simulink model "quadrotor_r2022b"  (R2022b)
settings: Solver=ode4  StartTime=0.0  StopTime=60  FixedStep=1e-3  RelTol=1e-3
libraries: slpidlib x10, dspindex x6, sharedtransform x3, simulink x3, shared6dof x1
(part 1 of 2)
Description:
  | 22
settings Model: Creator=vplus  LastModifiedBy=vplus

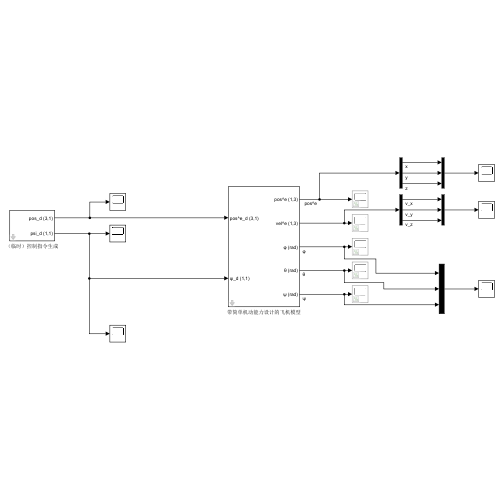
[thumbnail: Simulink's stored preview of the top-level diagram]
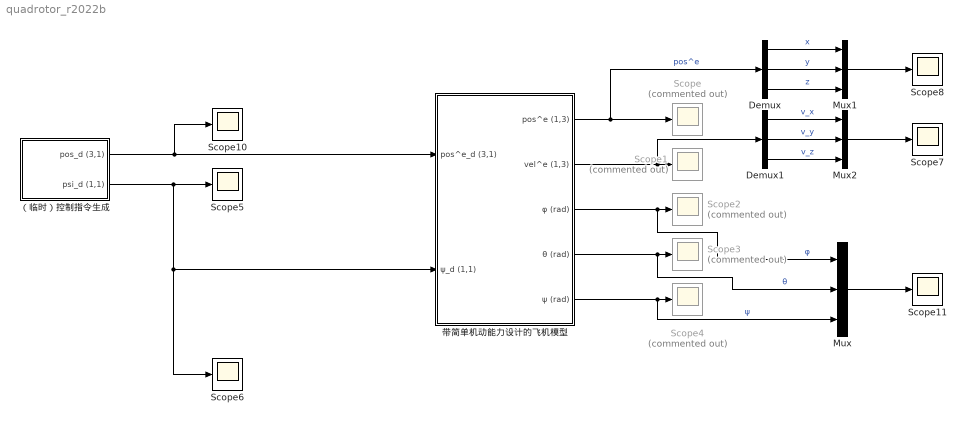
== system quadrotor_r2022b ==
  Demux : Demux  Outputs=3
  Demux1 : Demux  Outputs=3
  Mux : Mux  Inputs=3
  Mux1 : Mux  Inputs=3
  Mux2 : Mux  Inputs=3
  Scope{,1..4} (5 alike) : Scope  Commented=on
  Scope{5..8,10..11} (6 alike) : Scope
  带简单机动能力设计的飞机模型 : Subsystem  mask{Delta_t_theta=2.0, alpha_G=0.01, beta_G=0.5, rotor_w_max_rpm=240, n_rotors=4, g=9.8, mass=1.0, innertia=eye(3)}
      mask prompts: Delta_t_theta "转90° 预期时间 Δt_θ (s)"; alpha_G "α_G"; beta_G "β_G"; rotor_w_max_rpm "单发最大转速 ω_max (r/min)"; n_rotors "旋翼个数 n"; g "重力加速度 g (m/s^2)"; mass "质量 m (kg)"; innertia "转动惯量矩阵 I (kg*m^2)"
      mask init:
      | rpm2radps = (2*pi/60);
      | rotor_w_max = rotor_w_max_rpm*rpm2radps
      | % 拉力
      | f_max = (1+beta_G)*(mass*g);
      | C_T = f_max/(n_rotors* rotor_w_max^2)
      | rotor_w_min = rotor_w_max* sqrt((1-alpha_G)/(1+beta_G))
      | rotor_w_min_rpm = rotor_w_min/rpm2radps
      | 
      | % 角速度限制
      | dot_omega_z_max = 4*(pi/2)/(Delta_t_theta^2);
      | tau_z_max = abs(innertia(3,3)*dot_omega_z_max)
      | 
      | % 扭矩
      | C_M = tau_z_max/(2*(rotor_w_max^2-rotor_w_min^2))
      mask DialogControl ParameterGroupVar Prompt: 参数
      mask DialogControl Container3 Prompt: 拉力系数计算
  （临时）控制指令生成 : Subsystem  mask{rpy_0=[0,0,0], pos_0=[10,30,-2], vel_0=[1,1,0], a_h_max=1e-2, a_z_max=1e-3}
      mask prompts: rpy_0 "初始欧拉角 [φ,θ,ψ]_d (1,3) rad"; pos_0 "初始位置 p^e_d (1,3) (m/s)"; vel_0 "初始速度 v^e_d (1,3) (m/s)"; a_h_max "横向加速度最大值 a_h_max"; a_z_max "纵向加速度最大值 a_z_max"
      mask DialogControl ParameterGroupVar Prompt: 参数
  wires:
  Demux/1 -> Mux1/1  "x"
  Demux/3 -> Mux1/3  "z"
  Demux/2 -> Mux1/2  "y"
  （临时）控制指令生成/2(psi_d (1,1)) -> Scope5/1, 带简单机动能力设计的飞机模型/2("ψ_d (1,1) "), Scope6/1
  （临时）控制指令生成/1(pos_d (3,1)) -> 带简单机动能力设计的飞机模型/1(pos^e_d (3,1)), Scope10/1
  带简单机动能力设计的飞机模型/1(pos^e (1,3)) -> Demux/1, Scope/1  "pos^e"
  带简单机动能力设计的飞机模型/3(φ (rad)) -> Mux/1, Scope2/1  "φ"
  带简单机动能力设计的飞机模型/4(θ (rad)) -> Mux/2, Scope3/1  "θ"
  带简单机动能力设计的飞机模型/5(ψ (rad)) -> Mux/3, Scope4/1  "ψ"
  Mux/1 -> Scope11/1
  Mux1/1 -> Scope8/1
  Demux1/3 -> Mux2/3  "v_z"
  Mux2/1 -> Scope7/1
  带简单机动能力设计的飞机模型/2(vel^e (1,3)) -> Demux1/1, Scope1/1
  Demux1/2 -> Mux2/2  "v_y"
  Demux1/1 -> Mux2/1  "v_x"

== system quadrotor_r2022b/带简单机动能力设计的飞机模型 ==
  pos^e_d (3,1) : Inport
  "ψ_d (1,1) " : Inport  Port=2
  四旋翼无人机 : Subsystem  mask{mass=mass, innertia=innertia, g=g, C_T=C_T, C_M=C_M, L=0.2, w_max_rpm=rotor_w_max_rpm, w_min_rpm=rotor_w_min_rpm, pos_0_e=[0,0,0], vel_0_e=[0,0,0], rpy_0=[0,0,0], omega_0_b=[0,0,0], w_0=rotor_w_min*ones(1,4)}
      mask prompts: mass "质量 m (kg)"; innertia "体轴系转动惯量 I^b (kg*m^2)"; g "重力加速度 g  (m/s^2)"; C_T "旋翼拉力系数 C_T  (|T_i|=C_T*w_i^2)"; C_M "旋翼扭矩系数 C_M  (|M_i|=C_M*w_i^2)"; L "转子到体轴系原点的距离 L (m)"; w_max_rpm "旋翼最大转速 (r/min)"; w_min_rpm "旋翼最小转速 (r/min)"; pos_0_e "初始ned位置 p_0 (1,3) m"; vel_0_e "初始ned速度 v_0 (1,3) m/s"; rpy_0 "初始欧拉角 [φ,θ,ψ] (1,3) rad"; omega_0_b "初始角速度 ω^b (1,3) rad/s"; w_0 "初始旋翼转速 w (1,4) rad/s"
      mask init:
      | rpm2radps = 2*pi/60;
      | rotor_w_max = w_max_rpm *rpm2radps;
      | rotor_w_min = w_min_rpm *rpm2radps;
      | 
      | g_b = [0,0,1];
      | e_g_b = (g_b(:)/norm(g_b)); % 体轴系的重力方向,(3,1)
      | 
      | rotors_dir = [1,-1,1,-1];%旋翼的旋转方向(与体轴系Z同向记为正)
      | rotors_pos_b = [
      |     -1,-1,0;
      |     -1,1,0;
      |     1,1,0;
      |     1,-1,0
      | ]*L;% 四个旋翼的体轴系位置
      | 
      | rotors_dir=sign(rotors_dir(:)); % (n,1)
      | rotors_n = size(rotors_pos_b,1); % 电机数量
      | omegas=rotors_dir*(e_g_b'); % (n,3) 旋翼组的角速度朝向(右手定则,与重力同向为正)
      | 
      | assert(all(size(rotors_pos_b)==[rotors_n,3]),"旋翼相对位置格式错误")
      | assert(all(size(rotors_dir)==[rotors_n,1]),"旋翼旋转方向格式错误")
      | assert(all(size(e_g_b)==[3,1]),"重力方向尺寸错误")
      | 
      | f_max = rotors_n*C_T*(rotor_w_max^2); % 最大拉力
      | f_min = rotors_n*C_T*(rotor_w_min^2); % 最小拉力
      | mat_control=zeros(4,rotors_n); % [T,tau]=M*ws
      | for i=1:rotors_n
      | 
      |     r_i = rotors_pos_b(i,:);
      |     c_T_i = C_T*-e_g_b';
      | 
      |     c_MT_i = cross(r_i,c_T_i);
      |     c_MR_i = -C_M*omegas(i,:);
      |     c_M_i = c_MT_i + c_MR_i;
      |     for k=1:4
      |         if k==1
      |             mat_control(k,i) = -c_T_i(3);
      |         else
      |             mat_control(k,i) = c_M_i(k-1);
      |         end
      |     end
      | end
      | mat_control_inv = inv(mat_control);
      mask DialogControl DescTextVar Prompt: 体轴系为NED体轴系
      mask DialogControl ParameterGroupVar Prompt: 参数
      mask DialogControl Container3 Prompt: 初始状态
  pos^e (1,3) : Outport
  vel^e (1,3) : Outport  Port=2
  φ (rad) : Outport  Port=3
  θ (rad) : Outport  Port=4
  ψ (rad) : Outport  Port=5
  wires:
  "ψ_d (1,1) "/1 -> 四旋翼无人机/2("ψ_d (1,1) ")
  pos^e_d (3,1)/1 -> 四旋翼无人机/1(pos^e_d (3,1))
  四旋翼无人机/1(pos^e (1,3)) -> pos^e (1,3)/1  "pos^e"
  四旋翼无人机/2(vel^e (1,3)) -> vel^e (1,3)/1
  四旋翼无人机/3(φ (rad)) -> φ (rad)/1  "φ"
  四旋翼无人机/5(ψ (rad)) -> ψ (rad)/1  "ψ"
  四旋翼无人机/4(θ (rad)) -> θ (rad)/1  "θ"

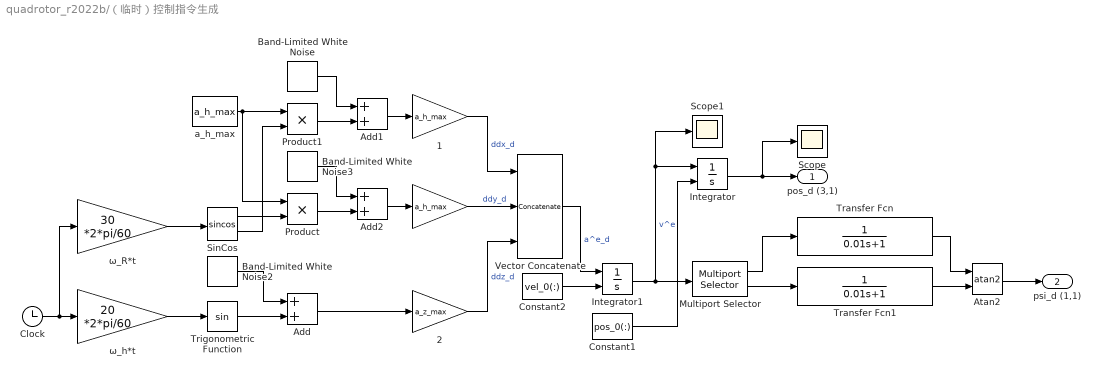
== system quadrotor_r2022b/（临时）控制指令生成 ==
  " " : Gain  Gain=a_h_max
  " 1" : Gain  Gain=a_h_max
  " 2" : Gain  Gain=a_z_max
  Add : Sum
  Add1 : Sum
  Add2 : Sum
  Atan2 : Trigonometry  Operator=atan2
  Band-Limited White Noise : simulink/Sources/Band-Limited White Noise  Cov=0.1  Ts=0.1  seed=[randi(10086)]
  Band-Limited White Noise2 : simulink/Sources/Band-Limited White Noise  Cov=0.1  Ts=0.1  seed=[randi(10086)]
  Band-Limited White Noise3 : simulink/Sources/Band-Limited White Noise  Cov=0.1  Ts=0.1  seed=[randi(10086)]
  Clock : Clock
  Constant1 : Constant  Value=pos_0(:)  VectorParams1D=off
  Constant2 : Constant  Value=vel_0(:)  VectorParams1D=off
  Integrator : Integrator  InitialConditionSource=external
  Integrator1 : Integrator  InitialConditionSource=external
  Multiport Selector : dspindex/Multiport Selector  rowsOrCols=Rows  idxCellArray={2,1}  idxErrMode=Clip Index
  Product : Product
  Product1 : Product
  Scope : Scope
  Scope1 : Scope
  SinCos : Trigonometry  Operator=sincos
  Transfer Fcn : TransferFcn  Denominator=[0.01 1]
  Transfer Fcn1 : TransferFcn  Denominator=[0.01 1]
  Trigonometric Function : Trigonometry
  Vector Concatenate : Concatenate  NumInputs=3  Mode=Multidimensional array
  a_h_max : Constant  Value=a_h_max  VectorParams1D=off
  ω_R*t : Gain  Gain=30 *2*pi/60
  ω_h*t : Gain  Gain=20 *2*pi/60
  pos_d (3,1) : Outport
  psi_d (1,1) : Outport  Port=2
  wires:
  Add1/1 -> " 1"/1
  SinCos/2 -> Product1/2
  SinCos/1 -> Product/2
  Clock/1 -> ω_R*t/1, ω_h*t/1
  ω_R*t/1 -> SinCos/1
  ω_h*t/1 -> Trigonometric Function/1
  Band-Limited White Noise/1 -> Add1/1
  Trigonometric Function/1 -> Add/2
  Constant2/1 -> Integrator1/2
  a_h_max/1 -> Product/1, Product1/1
  Product/1 -> Add2/2
  Band-Limited White Noise2/1 -> Add/1
  Product1/1 -> Add1/2
  Band-Limited White Noise3/1 -> Add2/1
  Add/1 -> " 2"/1
  Add2/1 -> " "/1
  " 1"/1 -> Vector Concatenate/1  "ddx_d"
  " "/1 -> Vector Concatenate/2  "ddy_d"
  " 2"/1 -> Vector Concatenate/3  "ddz_d"
  Vector Concatenate/1 -> Integrator1/1  "a^e_d"
  Integrator1/1 -> Integrator/1, Scope1/1, Multiport Selector/1  "v^e"
  Constant1/1 -> Integrator/2
  Integrator/1 -> pos_d (3,1)/1, Scope/1
  Multiport Selector/1 -> Transfer Fcn/1
  Multiport Selector/2 -> Transfer Fcn1/1
  Transfer Fcn/1 -> Atan2/1
  Transfer Fcn1/1 -> Atan2/2
  Atan2/1 -> psi_d (1,1)/1

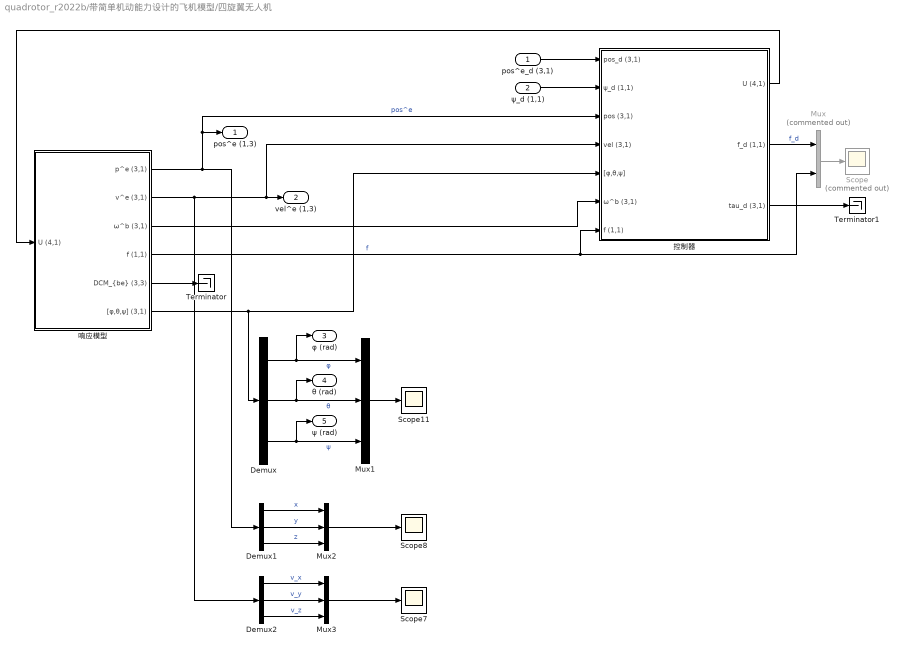
== system quadrotor_r2022b/带简单机动能力设计的飞机模型/四旋翼无人机 ==
  pos^e_d (3,1) : Inport
  "ψ_d (1,1) " : Inport  Port=2
  Demux : Demux  Outputs=3
  Demux1 : Demux  Outputs=3
  Demux2 : Demux  Outputs=3
  Mux : Mux  Commented=on  Inputs=2
  Mux1 : Mux  Inputs=3
  Mux2 : Mux  Inputs=3
  Mux3 : Mux  Inputs=3
  Scope : Scope  Commented=on
  Scope11 : Scope
  Scope7 : Scope
  Scope8 : Scope
  Terminator : Terminator
  Terminator1 : Terminator
  响应模型 : Subsystem
  控制器 : Subsystem
  pos^e (1,3) : Outport
  vel^e (1,3) : Outport  Port=2
  φ (rad) : Outport  Port=3
  θ (rad) : Outport  Port=4
  ψ (rad) : Outport  Port=5
  wires:
  控制器/3(tau_d (3,1)) -> Terminator1/1
  响应模型/4(f (1,1)) -> Mux/2, 控制器/7(f (1,1))  "f"
  响应模型/6("[φ,θ,ψ] (3,1)") -> 控制器/5("[φ,θ,ψ]"), Demux/1
  pos^e_d (3,1)/1 -> 控制器/1(pos_d (3,1))
  "ψ_d (1,1) "/1 -> 控制器/2(ψ_d (1,1))
  Mux/1 -> Scope/1
  响应模型/3(ω^b (3,1)) -> 控制器/6(ω^b (3,1))
  控制器/1(U (4,1)) -> 响应模型/1(U (4,1))
  控制器/2(f_d (1,1)) -> Mux/1  "f_d"
  响应模型/5("DCM_{be} (3,3)") -> Terminator/1
  Demux/1 -> Mux1/1, φ (rad)/1  "φ"
  Demux/3 -> ψ (rad)/1, Mux1/3  "ψ"
  Demux2/2 -> Mux3/2  "v_y"
  Demux2/3 -> Mux3/3  "v_z"
  Demux2/1 -> Mux3/1  "v_x"
  Mux2/1 -> Scope8/1
  Mux3/1 -> Scope7/1
  Demux1/3 -> Mux2/3  "z"
  Demux1/1 -> Mux2/1  "x"
  Mux1/1 -> Scope11/1
  Demux/2 -> Mux1/2, θ (rad)/1  "θ"
  响应模型/1(" p^e (3,1)") -> Demux1/1, 控制器/3(pos (3,1)), pos^e (1,3)/1  "pos^e"
  Demux1/2 -> Mux2/2  "y"
  响应模型/2(v^e (3,1)) -> Demux2/1, 控制器/4(vel (3,1)), vel^e (1,3)/1

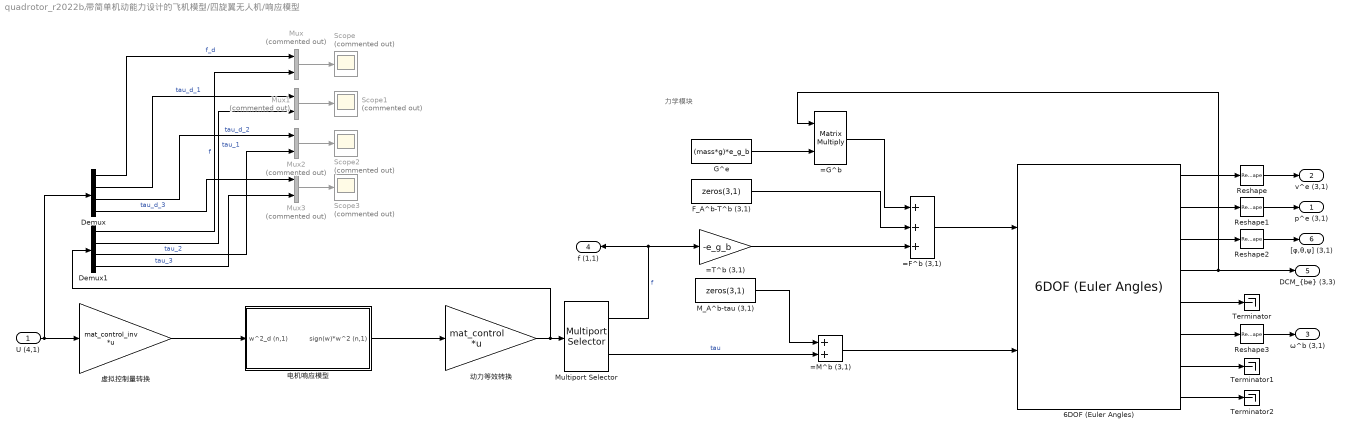
== system quadrotor_r2022b/带简单机动能力设计的飞机模型/四旋翼无人机/响应模型 ==
  note: 力学模块
  U (4,1) : Inport
  6DOF (Euler Angles) : shared6dof/6DOF (Euler Angles)  units=Metric (MKS)  mtype=Fixed  rep=Euler Angles  xme_0=pos_0_e(:)'  Vm_0=vel_0_e(:)'  eul_0=rpy_0(:)'  pm_0=omega_0_b(:)'  mass_0=mass  mass_e=0.5  mass_f=2.0  inertia=innertia  inertia_e=eye(3)  inertia_f=2*eye(3)  k_quat=1.0  vre_flag=on  abi_flag=off  aMode=0  xme_statename=''  Vm_statename=''  eul_statename=''  quat_statename=''  pm_statename=''  mass_statename=''
      settings: AttributesFormatString=DCM_{be}=R_{e_1,-roll}*R_{e_2,-pitch}*R_{e_3,-yaw}
  =F^b (3,1) : Sum  Inputs=+++
  =G^b : Product  Multiplication=Matrix(*)
  =M^b (3,1) : Sum
  =T^b (3,1) : Gain  Gain=-e_g_b
  Demux : Demux
  Demux1 : Demux
  F_A^b-T^b (3,1) : Constant  Value=zeros(3,1)  VectorParams1D=off
      settings: AttributesFormatString=其他气动力
  G^e : Constant  Value=(mass*g)*e_g_b  VectorParams1D=off
  M_A^b-tau (3,1) : Constant  Value=zeros(3,1)  VectorParams1D=off
      settings: AttributesFormatString=其他气动力矩
  Multiport Selector : dspindex/Multiport Selector  rowsOrCols=Rows  idxCellArray={1,2:4}  idxErrMode=Clip Index
  Mux{,1..3} (4 alike) : Mux  Commented=on  Inputs=2
  Reshape{,1..3} (4 alike) : Reshape  OutputDimensionality=Column vector (2-D)
  Scope{,1..3} (4 alike) : Scope  Commented=on
  Terminator : Terminator
  Terminator1 : Terminator
  Terminator2 : Terminator
  动力等效转换 : Gain  Gain=mat_control  Multiplication=Matrix(K*u)
  电机响应模型 : Subsystem  mask{tau=0.2}
      mask prompts: tau "电机延迟系数 τ"
      mask DialogControl ParameterGroupVar Prompt: 参数
  虚拟控制量转换 : Gain  Gain=mat_control_inv  Multiplication=Matrix(K*u)
  " p^e (3,1)" : Outport
  v^e (3,1) : Outport  Port=2
  ω^b (3,1) : Outport  Port=3
  f (1,1) : Outport  Port=4
  "DCM_{be} (3,3)" : Outport  Port=5
  "[φ,θ,ψ] (3,1)" : Outport  Port=6
  wires:
  =T^b (3,1)/1 -> =F^b (3,1)/3
  电机响应模型/1(sign(w)*w^2 (n,1)) -> 动力等效转换/1
  U (4,1)/1 -> Demux/1, 虚拟控制量转换/1
  Multiport Selector/1 -> f (1,1)/1, =T^b (3,1)/1  "f"
  6DOF (Euler Angles)/1 -> Reshape/1
  6DOF (Euler Angles)/2 -> Reshape1/1
  6DOF (Euler Angles)/3 -> Reshape2/1
  6DOF (Euler Angles)/5 -> Terminator/1
  6DOF (Euler Angles)/4 -> "DCM_{be} (3,3)"/1, =G^b/1
  6DOF (Euler Angles)/6 -> Reshape3/1
  6DOF (Euler Angles)/8 -> Terminator2/1
  6DOF (Euler Angles)/7 -> Terminator1/1
  =M^b (3,1)/1 -> 6DOF (Euler Angles)/2
  G^e/1 -> =G^b/2
  =F^b (3,1)/1 -> 6DOF (Euler Angles)/1
  =G^b/1 -> =F^b (3,1)/1
  F_A^b-T^b (3,1)/1 -> =F^b (3,1)/2
  Multiport Selector/2 -> =M^b (3,1)/2  "tau"
  M_A^b-tau (3,1)/1 -> =M^b (3,1)/1
  Reshape/1 -> v^e (3,1)/1
  Reshape1/1 -> " p^e (3,1)"/1
  Reshape2/1 -> "[φ,θ,ψ] (3,1)"/1
  Reshape3/1 -> ω^b (3,1)/1
  动力等效转换/1 -> Demux1/1, Multiport Selector/1
  虚拟控制量转换/1 -> 电机响应模型/1(w^2_d (n,1))
  Mux/1 -> Scope/1
  Demux/1 -> Mux/1  "f_d"
  Demux1/1 -> Mux/2  "f"
  Demux/2 -> Mux1/1  "tau_d_1"
  Demux1/2 -> Mux1/2  "tau_1"
  Mux1/1 -> Scope1/1
  Demux1/3 -> Mux2/2  "tau_2"
  Demux/3 -> Mux2/1  "tau_d_2"
  Mux2/1 -> Scope2/1
  Demux1/4 -> Mux3/2  "tau_3"
  Demux/4 -> Mux3/1  "tau_d_3"
  Mux3/1 -> Scope3/1

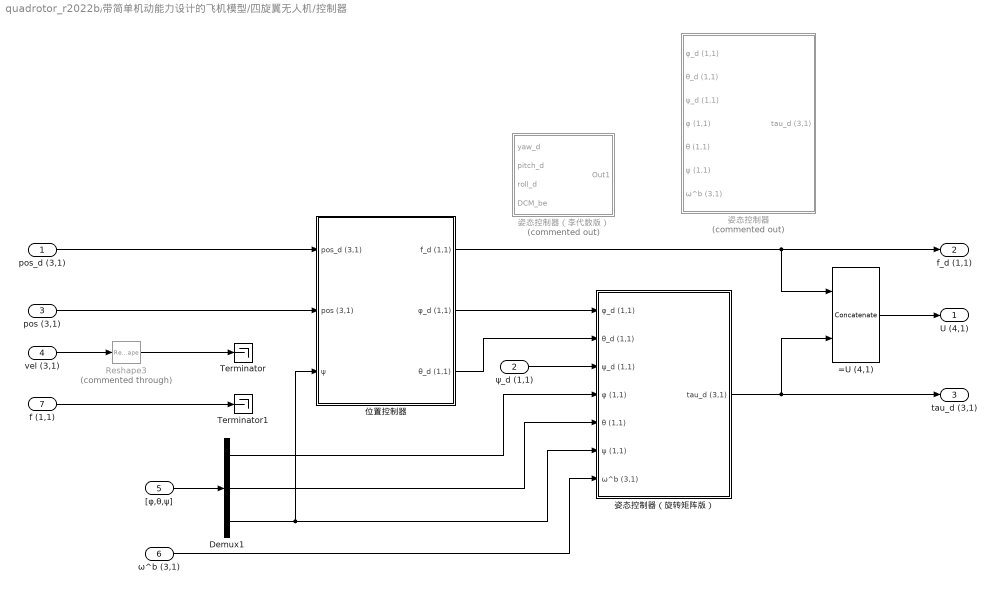
== system quadrotor_r2022b/带简单机动能力设计的飞机模型/四旋翼无人机/控制器 ==
  pos_d (3,1) : Inport
  ψ_d (1,1) : Inport  Port=2
  pos (3,1) : Inport  Port=3
  vel (3,1) : Inport  Port=4
  "[φ,θ,ψ]" : Inport  Port=5
  ω^b (3,1) : Inport  Port=6
  f (1,1) : Inport  Port=7
  =U (4,1) : Concatenate  Mode=Multidimensional array
  Demux1 : Demux  Outputs=3
  Reshape3 : Reshape  Commented=through  OutputDimensionality=Column vector (2-D)
  Terminator : Terminator
  Terminator1 : Terminator
  位置控制器 : Subsystem  mask{K_P_h=0.0058932, K_D_h=0.71637, K_N_h=10.3468, K_P_z=0.65677, K_D_z=2.1365, K_N_z=191.796}
      mask prompts: K_P_h "K_{P,p_h}"; K_D_h "K_{D,p_h}"; K_N_h "K_{N,p_h}"; K_P_z "K_{P,p_z}"; K_D_z "K_{D,p_z}"; K_N_z "K_{N,p_z}"
      mask init:
      | A_ange2vel = [];
      mask DialogControl ParameterGroupVar Prompt: 水平通道PID参数
      mask DialogControl Container3 Prompt: 纵向通道PID参数
  姿态控制器 : Subsystem  Commented=on  mask{K_R=0.1, K_w=0.1}
      mask DialogControl ParameterGroupVar Prompt: 参数
  姿态控制器（旋转矩阵版） : Subsystem  mask{K_R=2.0, K_w=8.0}
      mask DialogControl ParameterGroupVar Prompt: 参数
  姿态控制器（李代数版） : Subsystem  Commented=on
  U (4,1) : Outport
  f_d (1,1) : Outport  Port=2
  tau_d (3,1) : Outport  Port=3
  wires:
  "[φ,θ,ψ]"/1 -> Demux1/1
  vel (3,1)/1 -> Reshape3/1
  f (1,1)/1 -> Terminator1/1
  Demux1/3 -> 姿态控制器（旋转矩阵版）/6(ψ (1,1)), 位置控制器/3(ψ)
  位置控制器/2(φ_d (1,1)) -> 姿态控制器（旋转矩阵版）/1(φ_d (1,1))
  位置控制器/3(θ_d (1,1)) -> 姿态控制器（旋转矩阵版）/2(θ_d (1,1))
  ψ_d (1,1)/1 -> 姿态控制器（旋转矩阵版）/3(ψ_d (1,1))
  pos_d (3,1)/1 -> 位置控制器/1(pos_d (3,1))
  pos (3,1)/1 -> 位置控制器/2(pos (3,1))
  ω^b (3,1)/1 -> 姿态控制器（旋转矩阵版）/7(ω^b (3,1))
  =U (4,1)/1 -> U (4,1)/1
  Reshape3/1 -> Terminator/1
  姿态控制器（旋转矩阵版）/1(tau_d (3,1)) -> =U (4,1)/2, tau_d (3,1)/1
  位置控制器/1(f_d (1,1)) -> =U (4,1)/1, f_d (1,1)/1
  Demux1/2 -> 姿态控制器（旋转矩阵版）/5(θ (1,1))
  Demux1/1 -> 姿态控制器（旋转矩阵版）/4(φ (1,1))

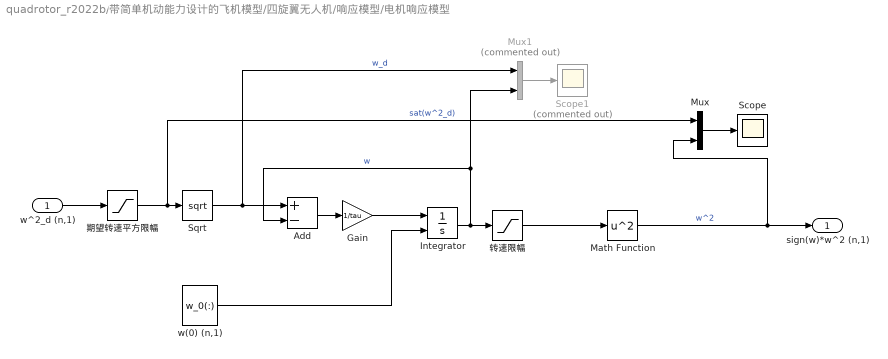
== system quadrotor_r2022b/带简单机动能力设计的飞机模型/四旋翼无人机/响应模型/电机响应模型 ==
  w^2_d (n,1) : Inport
  Add : Sum  Inputs=+-
  Gain : Gain  Gain=1/tau
  Integrator : Integrator  InitialConditionSource=external
  Math Function : Math  Operator=square
  Mux : Mux  Inputs=2
  Mux1 : Mux  Commented=on  Inputs=2
  Scope : Scope
  Scope1 : Scope  Commented=on
  Sqrt : Sqrt  OutputSignalType=real
  w(0) (n,1) : Constant  Value=w_0(:)  VectorParams1D=off
  期望转速平方限幅 : Saturate  UpperLimit=rotor_w_max^2  LowerLimit=rotor_w_min^2
  转速限幅 : Saturate  UpperLimit=rotor_w_max  LowerLimit=rotor_w_min  ZeroCross=off
  sign(w)*w^2 (n,1) : Outport
  wires:
  转速限幅/1 -> Math Function/1
  w^2_d (n,1)/1 -> 期望转速平方限幅/1
  Add/1 -> Gain/1
  Gain/1 -> Integrator/1
  Mux/1 -> Scope/1
  期望转速平方限幅/1 -> Mux/1, Sqrt/1  "sat(w^2_d)"
  w(0) (n,1)/1 -> Integrator/2
  Integrator/1 -> Mux1/2, Add/2, 转速限幅/1  "w"
  Math Function/1 -> sign(w)*w^2 (n,1)/1, Mux/2  "w^2"
  Sqrt/1 -> Add/1, Mux1/1  "w_d"
  Mux1/1 -> Scope1/1

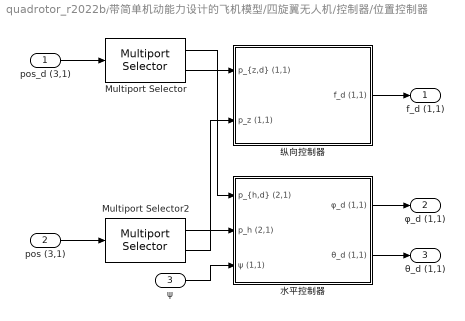
== system quadrotor_r2022b/带简单机动能力设计的飞机模型/四旋翼无人机/控制器/位置控制器 ==
  pos_d (3,1) : Inport
  pos (3,1) : Inport  Port=2
  ψ : Inport  Port=3
  Multiport Selector : dspindex/Multiport Selector  rowsOrCols=Rows  idxCellArray={1:2,3}  idxErrMode=Clip Index
  Multiport Selector2 : dspindex/Multiport Selector  rowsOrCols=Rows  idxCellArray={1:2,3}  idxErrMode=Clip Index
  水平控制器 : Subsystem
  纵向控制器 : Subsystem
  f_d (1,1) : Outport
  φ_d (1,1) : Outport  Port=2
  θ_d (1,1) : Outport  Port=3
  wires:
  Multiport Selector2/2 -> 纵向控制器/2(p_z (1,1))
  纵向控制器/1(f_d (1,1)) -> f_d (1,1)/1
  Multiport Selector2/1 -> 水平控制器/2(p_h (2,1))
  pos_d (3,1)/1 -> Multiport Selector/1
  ψ/1 -> 水平控制器/3(ψ (1,1))
  pos (3,1)/1 -> Multiport Selector2/1
  Multiport Selector/2 -> 纵向控制器/1("p_{z,d} (1,1)")
  Multiport Selector/1 -> 水平控制器/1("p_{h,d} (2,1)")
  水平控制器/1(φ_d (1,1)) -> φ_d (1,1)/1
  水平控制器/2(θ_d (1,1)) -> θ_d (1,1)/1

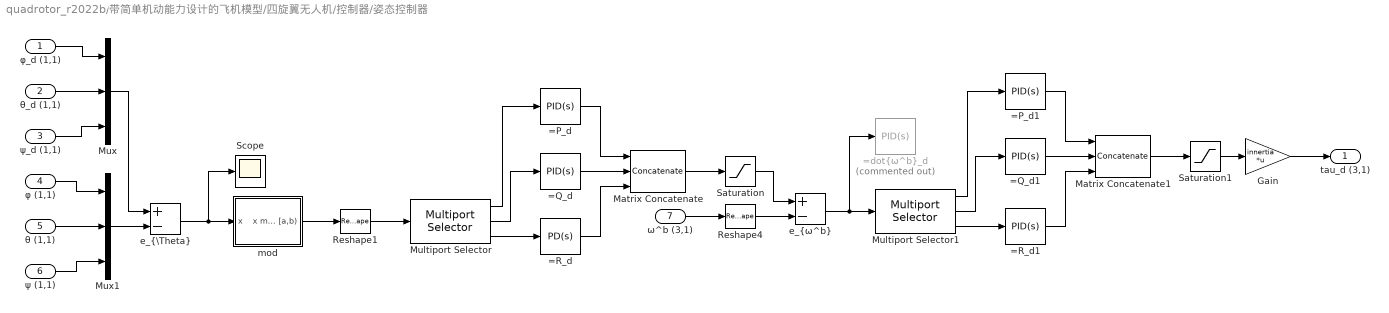
== system quadrotor_r2022b/带简单机动能力设计的飞机模型/四旋翼无人机/控制器/姿态控制器 ==
  φ_d (1,1) : Inport
  θ_d (1,1) : Inport  Port=2
  ψ_d (1,1) : Inport  Port=3
  φ (1,1) : Inport  Port=4
  θ (1,1) : Inport  Port=5
  ψ (1,1) : Inport  Port=6
  ω^b (3,1) : Inport  Port=7
  =P_d : slpidlib/PID Controller  Controller=PID  Form=Parallel  TimeDomain=Continuous-time  UseExternalTs=off  SampleTime=-1  IntegratorMethod=Forward Euler  FilterMethod=Forward Euler  ControllerParametersSource=internal  P=0.1  I=0  UseKiTs=off  D=0  N=100  UseFilter=on  TunerSelectOption=Frequency Response Based  InitialConditionSource=internal  InitialConditionForIntegrator=0  InitialConditionForFilter=0  DifferentiatorICPrevScaledInput=0  ExternalReset=none  TrackingMode=off  Kt=1  LimitOutput=off  SatLimitsSource=internal  UpperSaturationLimit=inf  LowerSaturationLimit=-inf  LinearizeAsGain=on  AntiWindupMode=none  Kb=1  LimitIntegrator=off  UpperIntegratorSaturationLimit=inf  LowerIntegratorSaturationLimit=-inf  POutMin=[]  POutMax=[]  IOutMin=[]  IOutMax=[]  DOutMin=[]  DOutMax=[]  NOutMin=[]  NOutMax=[]  SumOutMin=[]  SumOutMax=[]  SaturationOutMin=[]  SaturationOutMax=[]  PParamMin=[]  PParamMax=[]  IParamMin=[]  IParamMax=[]  DParamMin=[]  DParamMax=[]  NParamMin=[]  NParamMax=[]  KbParamMin=[]  KbParamMax=[]  KtParamMin=[]  KtParamMax=[]  KbOutMin=[]  KbOutMax=[]  KtOutMin=[]  KtOutMax=[]  IntegratorOutMin=[]  IntegratorOutMax=[]  FilterOutMin=[]  FilterOutMax=[]  SumI1OutMin=[]  SumI1OutMax=[]  SumI2OutMin=[]  SumI2OutMax=[]  SumI3OutMin=[]  SumI3OutMax=[]  SumI4OutMin=[]  SumI4OutMax=[]  SumDOutMin=[]  SumDOutMax=[]  DifferentiatorOutMin=[]  DifferentiatorOutMax=[]  FilterDiffOutCoefMin=[]  FilterDiffOutCoefMax=[]  ReciprocalOutMin=[]  ReciprocalOutMax=[]  SumDenOutMin=[]  SumDenOutMax=[]  SumNumOutMin=[]  SumNumOutMax=[]  DivideOutMin=[]  DivideOutMax=[]  UdiffTsProdOutMin=[]  UdiffTsProdOutMax=[]  NTsProdOutMin=[]  NTsProdOutMax=[]  UintegralTsProdOutMin=[]  UintegralTsProdOutMax=[]  UngainTsProdOutMin=[]  UngainTsProdOutMax=[]  ClampingZeroOutDataTypeStr=Inherit: Inherit via back propagation  ClampingZeroOutMin=[]  ClampingZeroOutMax=[]  FilterDenConstantOutDataTypeStr=Inherit: Inherit via back propagation  FilterDenConstantOutMin=[]  FilterDenConstantOutMax=[]  PCopyOutDataTypeStr=Inherit: Inherit via back propagation  PCopyOutMin=[]  PCopyOutMax=[]  NCopyOutDataTypeStr=Inherit: Inherit via back propagation  NCopyOutMin=[]  NCopyOutMax=[]  IntegratorContinuousStateAttributes=''  IntegratorStateMustResolveToSignalObject=off  IntegratorRTWStateStorageClass=Auto  FilterContinuousStateAttributes=''  FilterStateMustResolveToSignalObject=off  FilterRTWStateStorageClass=Auto  ParallelPVariant=InternalParameters  IdealPVariant=Disabled  IVariant=InternalParameters  DVariant=InternalParameters  IntegratorVariant=Continuous  SatVariant=Disabled  AWVariant=Passthrough  PCopyVariant=Disabled  TRVariant=Disabled  FdbkBlocksVariant=Forward  IdealPFdbkVariant=Disabled  SatFdbkVariant=Disabled  DerivativeFilterVariant=ContFilter  NVariant=InternalParameters  NCopyVariant=Disabled  FilterICVariant=InternalICsFilter  IntegratorICVariant=InternalICs  ExternalResetVariant=Disabled  TRSumVariant=Passthrough  SumFdbkVariant=Disabled  SumVariant=Sum_PID  TsampFilterVariant=InternalTs  TsampNgainVariant=Passthrough  TsampIntegralVariant=Passthrough  ExternalSaturationOutDataTypeStr=Inherit: Same as second input
  =P_d1 : slpidlib/PID Controller  Controller=PID  Form=Parallel  TimeDomain=Continuous-time  UseExternalTs=off  SampleTime=-1  IntegratorMethod=Forward Euler  FilterMethod=Forward Euler  ControllerParametersSource=internal  P=0.1  I=0  UseKiTs=off  D=0  N=100  UseFilter=on  TunerSelectOption=Transfer Function Based (PID Tuner App)  InitialConditionSource=internal  InitialConditionForIntegrator=0  InitialConditionForFilter=0  DifferentiatorICPrevScaledInput=0  ExternalReset=none  TrackingMode=off  Kt=1  LimitOutput=off  SatLimitsSource=internal  UpperSaturationLimit=inf  LowerSaturationLimit=-inf  LinearizeAsGain=on  AntiWindupMode=none  Kb=1  LimitIntegrator=off  UpperIntegratorSaturationLimit=inf  LowerIntegratorSaturationLimit=-inf  POutMin=[]  POutMax=[]  IOutMin=[]  IOutMax=[]  DOutMin=[]  DOutMax=[]  NOutMin=[]  NOutMax=[]  SumOutMin=[]  SumOutMax=[]  SaturationOutMin=[]  SaturationOutMax=[]  PParamMin=[]  PParamMax=[]  IParamMin=[]  IParamMax=[]  DParamMin=[]  DParamMax=[]  NParamMin=[]  NParamMax=[]  KbParamMin=[]  KbParamMax=[]  KtParamMin=[]  KtParamMax=[]  KbOutMin=[]  KbOutMax=[]  KtOutMin=[]  KtOutMax=[]  IntegratorOutMin=[]  IntegratorOutMax=[]  FilterOutMin=[]  FilterOutMax=[]  SumI1OutMin=[]  SumI1OutMax=[]  SumI2OutMin=[]  SumI2OutMax=[]  SumI3OutMin=[]  SumI3OutMax=[]  SumI4OutMin=[]  SumI4OutMax=[]  SumDOutMin=[]  SumDOutMax=[]  DifferentiatorOutMin=[]  DifferentiatorOutMax=[]  FilterDiffOutCoefMin=[]  FilterDiffOutCoefMax=[]  ReciprocalOutMin=[]  ReciprocalOutMax=[]  SumDenOutMin=[]  SumDenOutMax=[]  SumNumOutMin=[]  SumNumOutMax=[]  DivideOutMin=[]  DivideOutMax=[]  UdiffTsProdOutMin=[]  UdiffTsProdOutMax=[]  NTsProdOutMin=[]  NTsProdOutMax=[]  UintegralTsProdOutMin=[]  UintegralTsProdOutMax=[]  UngainTsProdOutMin=[]  UngainTsProdOutMax=[]  ClampingZeroOutDataTypeStr=Inherit: Inherit via back propagation  ClampingZeroOutMin=[]  ClampingZeroOutMax=[]  FilterDenConstantOutDataTypeStr=Inherit: Inherit via back propagation  FilterDenConstantOutMin=[]  FilterDenConstantOutMax=[]  PCopyOutDataTypeStr=Inherit: Inherit via back propagation  PCopyOutMin=[]  PCopyOutMax=[]  NCopyOutDataTypeStr=Inherit: Inherit via back propagation  NCopyOutMin=[]  NCopyOutMax=[]  IntegratorContinuousStateAttributes=''  IntegratorStateMustResolveToSignalObject=off  IntegratorRTWStateStorageClass=Auto  FilterContinuousStateAttributes=''  FilterStateMustResolveToSignalObject=off  FilterRTWStateStorageClass=Auto  ParallelPVariant=InternalParameters  IdealPVariant=Disabled  IVariant=InternalParameters  DVariant=InternalParameters  IntegratorVariant=Continuous  SatVariant=Disabled  AWVariant=Passthrough  PCopyVariant=Disabled  TRVariant=Disabled  FdbkBlocksVariant=Forward  IdealPFdbkVariant=Disabled  SatFdbkVariant=Disabled  DerivativeFilterVariant=ContFilter  NVariant=InternalParameters  NCopyVariant=Disabled  FilterICVariant=InternalICsFilter  IntegratorICVariant=InternalICs  ExternalResetVariant=Disabled  TRSumVariant=Passthrough  SumFdbkVariant=Disabled  SumVariant=Sum_PID  TsampFilterVariant=InternalTs  TsampNgainVariant=Passthrough  TsampIntegralVariant=Passthrough  ExternalSaturationOutDataTypeStr=Inherit: Same as second input
  =Q_d : slpidlib/PID Controller  Controller=PID  Form=Parallel  TimeDomain=Continuous-time  UseExternalTs=off  SampleTime=-1  IntegratorMethod=Forward Euler  FilterMethod=Forward Euler  ControllerParametersSource=internal  P=0.1  I=0  UseKiTs=off  D=0  N=100  UseFilter=on  TunerSelectOption=Transfer Function Based (PID Tuner App)  InitialConditionSource=internal  InitialConditionForIntegrator=0  InitialConditionForFilter=0  DifferentiatorICPrevScaledInput=0  ExternalReset=none  TrackingMode=off  Kt=1  LimitOutput=off  SatLimitsSource=internal  UpperSaturationLimit=inf  LowerSaturationLimit=-inf  LinearizeAsGain=on  AntiWindupMode=none  Kb=1  LimitIntegrator=off  UpperIntegratorSaturationLimit=inf  LowerIntegratorSaturationLimit=-inf  POutMin=[]  POutMax=[]  IOutMin=[]  IOutMax=[]  DOutMin=[]  DOutMax=[]  NOutMin=[]  NOutMax=[]  SumOutMin=[]  SumOutMax=[]  SaturationOutMin=[]  SaturationOutMax=[]  PParamMin=[]  PParamMax=[]  IParamMin=[]  IParamMax=[]  DParamMin=[]  DParamMax=[]  NParamMin=[]  NParamMax=[]  KbParamMin=[]  KbParamMax=[]  KtParamMin=[]  KtParamMax=[]  KbOutMin=[]  KbOutMax=[]  KtOutMin=[]  KtOutMax=[]  IntegratorOutMin=[]  IntegratorOutMax=[]  FilterOutMin=[]  FilterOutMax=[]  SumI1OutMin=[]  SumI1OutMax=[]  SumI2OutMin=[]  SumI2OutMax=[]  SumI3OutMin=[]  SumI3OutMax=[]  SumI4OutMin=[]  SumI4OutMax=[]  SumDOutMin=[]  SumDOutMax=[]  DifferentiatorOutMin=[]  DifferentiatorOutMax=[]  FilterDiffOutCoefMin=[]  FilterDiffOutCoefMax=[]  ReciprocalOutMin=[]  ReciprocalOutMax=[]  SumDenOutMin=[]  SumDenOutMax=[]  SumNumOutMin=[]  SumNumOutMax=[]  DivideOutMin=[]  DivideOutMax=[]  UdiffTsProdOutMin=[]  UdiffTsProdOutMax=[]  NTsProdOutMin=[]  NTsProdOutMax=[]  UintegralTsProdOutMin=[]  UintegralTsProdOutMax=[]  UngainTsProdOutMin=[]  UngainTsProdOutMax=[]  ClampingZeroOutDataTypeStr=Inherit: Inherit via back propagation  ClampingZeroOutMin=[]  ClampingZeroOutMax=[]  FilterDenConstantOutDataTypeStr=Inherit: Inherit via back propagation  FilterDenConstantOutMin=[]  FilterDenConstantOutMax=[]  PCopyOutDataTypeStr=Inherit: Inherit via back propagation  PCopyOutMin=[]  PCopyOutMax=[]  NCopyOutDataTypeStr=Inherit: Inherit via back propagation  NCopyOutMin=[]  NCopyOutMax=[]  IntegratorContinuousStateAttributes=''  IntegratorStateMustResolveToSignalObject=off  IntegratorRTWStateStorageClass=Auto  FilterContinuousStateAttributes=''  FilterStateMustResolveToSignalObject=off  FilterRTWStateStorageClass=Auto  ParallelPVariant=InternalParameters  IdealPVariant=Disabled  IVariant=InternalParameters  DVariant=InternalParameters  IntegratorVariant=Continuous  SatVariant=Disabled  AWVariant=Passthrough  PCopyVariant=Disabled  TRVariant=Disabled  FdbkBlocksVariant=Forward  IdealPFdbkVariant=Disabled  SatFdbkVariant=Disabled  DerivativeFilterVariant=ContFilter  NVariant=InternalParameters  NCopyVariant=Disabled  FilterICVariant=InternalICsFilter  IntegratorICVariant=InternalICs  ExternalResetVariant=Disabled  TRSumVariant=Passthrough  SumFdbkVariant=Disabled  SumVariant=Sum_PID  TsampFilterVariant=InternalTs  TsampNgainVariant=Passthrough  TsampIntegralVariant=Passthrough  ExternalSaturationOutDataTypeStr=Inherit: Same as second input
  =Q_d1 : slpidlib/PID Controller  Controller=PID  Form=Parallel  TimeDomain=Continuous-time  UseExternalTs=off  SampleTime=-1  IntegratorMethod=Forward Euler  FilterMethod=Forward Euler  ControllerParametersSource=internal  P=0.1  I=0  UseKiTs=off  D=0  N=100  UseFilter=on  TunerSelectOption=Transfer Function Based (PID Tuner App)  InitialConditionSource=internal  InitialConditionForIntegrator=0  InitialConditionForFilter=0  DifferentiatorICPrevScaledInput=0  ExternalReset=none  TrackingMode=off  Kt=1  LimitOutput=off  SatLimitsSource=internal  UpperSaturationLimit=inf  LowerSaturationLimit=-inf  LinearizeAsGain=on  AntiWindupMode=none  Kb=1  LimitIntegrator=off  UpperIntegratorSaturationLimit=inf  LowerIntegratorSaturationLimit=-inf  POutMin=[]  POutMax=[]  IOutMin=[]  IOutMax=[]  DOutMin=[]  DOutMax=[]  NOutMin=[]  NOutMax=[]  SumOutMin=[]  SumOutMax=[]  SaturationOutMin=[]  SaturationOutMax=[]  PParamMin=[]  PParamMax=[]  IParamMin=[]  IParamMax=[]  DParamMin=[]  DParamMax=[]  NParamMin=[]  NParamMax=[]  KbParamMin=[]  KbParamMax=[]  KtParamMin=[]  KtParamMax=[]  KbOutMin=[]  KbOutMax=[]  KtOutMin=[]  KtOutMax=[]  IntegratorOutMin=[]  IntegratorOutMax=[]  FilterOutMin=[]  FilterOutMax=[]  SumI1OutMin=[]  SumI1OutMax=[]  SumI2OutMin=[]  SumI2OutMax=[]  SumI3OutMin=[]  SumI3OutMax=[]  SumI4OutMin=[]  SumI4OutMax=[]  SumDOutMin=[]  SumDOutMax=[]  DifferentiatorOutMin=[]  DifferentiatorOutMax=[]  FilterDiffOutCoefMin=[]  FilterDiffOutCoefMax=[]  ReciprocalOutMin=[]  ReciprocalOutMax=[]  SumDenOutMin=[]  SumDenOutMax=[]  SumNumOutMin=[]  SumNumOutMax=[]  DivideOutMin=[]  DivideOutMax=[]  UdiffTsProdOutMin=[]  UdiffTsProdOutMax=[]  NTsProdOutMin=[]  NTsProdOutMax=[]  UintegralTsProdOutMin=[]  UintegralTsProdOutMax=[]  UngainTsProdOutMin=[]  UngainTsProdOutMax=[]  ClampingZeroOutDataTypeStr=Inherit: Inherit via back propagation  ClampingZeroOutMin=[]  ClampingZeroOutMax=[]  FilterDenConstantOutDataTypeStr=Inherit: Inherit via back propagation  FilterDenConstantOutMin=[]  FilterDenConstantOutMax=[]  PCopyOutDataTypeStr=Inherit: Inherit via back propagation  PCopyOutMin=[]  PCopyOutMax=[]  NCopyOutDataTypeStr=Inherit: Inherit via back propagation  NCopyOutMin=[]  NCopyOutMax=[]  IntegratorContinuousStateAttributes=''  IntegratorStateMustResolveToSignalObject=off  IntegratorRTWStateStorageClass=Auto  FilterContinuousStateAttributes=''  FilterStateMustResolveToSignalObject=off  FilterRTWStateStorageClass=Auto  ParallelPVariant=InternalParameters  IdealPVariant=Disabled  IVariant=InternalParameters  DVariant=InternalParameters  IntegratorVariant=Continuous  SatVariant=Disabled  AWVariant=Passthrough  PCopyVariant=Disabled  TRVariant=Disabled  FdbkBlocksVariant=Forward  IdealPFdbkVariant=Disabled  SatFdbkVariant=Disabled  DerivativeFilterVariant=ContFilter  NVariant=InternalParameters  NCopyVariant=Disabled  FilterICVariant=InternalICsFilter  IntegratorICVariant=InternalICs  ExternalResetVariant=Disabled  TRSumVariant=Passthrough  SumFdbkVariant=Disabled  SumVariant=Sum_PID  TsampFilterVariant=InternalTs  TsampNgainVariant=Passthrough  TsampIntegralVariant=Passthrough  ExternalSaturationOutDataTypeStr=Inherit: Same as second input
  =R_d : slpidlib/PID Controller  Controller=PD  Form=Parallel  TimeDomain=Continuous-time  UseExternalTs=off  SampleTime=-1  IntegratorMethod=Forward Euler  FilterMethod=Forward Euler  ControllerParametersSource=internal  P=0.5  I=0  UseKiTs=off  D=0.5  N=100  UseFilter=on  TunerSelectOption=Transfer Function Based (PID Tuner App)  InitialConditionSource=internal  InitialConditionForIntegrator=0  InitialConditionForFilter=0  DifferentiatorICPrevScaledInput=0  ExternalReset=none  TrackingMode=off  Kt=1  LimitOutput=off  SatLimitsSource=internal  UpperSaturationLimit=inf  LowerSaturationLimit=-inf  LinearizeAsGain=on  AntiWindupMode=none  Kb=1  LimitIntegrator=off  UpperIntegratorSaturationLimit=inf  LowerIntegratorSaturationLimit=-inf  POutMin=[]  POutMax=[]  IOutMin=[]  IOutMax=[]  DOutMin=[]  DOutMax=[]  NOutMin=[]  NOutMax=[]  SumOutMin=[]  SumOutMax=[]  SaturationOutMin=[]  SaturationOutMax=[]  PParamMin=[]  PParamMax=[]  IParamMin=[]  IParamMax=[]  DParamMin=[]  DParamMax=[]  NParamMin=[]  NParamMax=[]  KbParamMin=[]  KbParamMax=[]  KtParamMin=[]  KtParamMax=[]  KbOutMin=[]  KbOutMax=[]  KtOutMin=[]  KtOutMax=[]  IntegratorOutMin=[]  IntegratorOutMax=[]  FilterOutMin=[]  FilterOutMax=[]  SumI1OutMin=[]  SumI1OutMax=[]  SumI2OutMin=[]  SumI2OutMax=[]  SumI3OutMin=[]  SumI3OutMax=[]  SumI4OutMin=[]  SumI4OutMax=[]  SumDOutMin=[]  SumDOutMax=[]  DifferentiatorOutMin=[]  DifferentiatorOutMax=[]  FilterDiffOutCoefMin=[]  FilterDiffOutCoefMax=[]  ReciprocalOutMin=[]  ReciprocalOutMax=[]  SumDenOutMin=[]  SumDenOutMax=[]  SumNumOutMin=[]  SumNumOutMax=[]  DivideOutMin=[]  DivideOutMax=[]  UdiffTsProdOutMin=[]  UdiffTsProdOutMax=[]  NTsProdOutMin=[]  NTsProdOutMax=[]  UintegralTsProdOutMin=[]  UintegralTsProdOutMax=[]  UngainTsProdOutMin=[]  UngainTsProdOutMax=[]  ClampingZeroOutDataTypeStr=Inherit: Inherit via back propagation  ClampingZeroOutMin=[]  ClampingZeroOutMax=[]  FilterDenConstantOutDataTypeStr=Inherit: Inherit via back propagation  FilterDenConstantOutMin=[]  FilterDenConstantOutMax=[]  PCopyOutDataTypeStr=Inherit: Inherit via back propagation  PCopyOutMin=[]  PCopyOutMax=[]  NCopyOutDataTypeStr=Inherit: Inherit via back propagation  NCopyOutMin=[]  NCopyOutMax=[]  IntegratorContinuousStateAttributes=''  IntegratorStateMustResolveToSignalObject=off  IntegratorRTWStateStorageClass=Auto  FilterContinuousStateAttributes=''  FilterStateMustResolveToSignalObject=off  FilterRTWStateStorageClass=Auto  ParallelPVariant=InternalParameters  IdealPVariant=Disabled  IVariant=Disabled  DVariant=InternalParameters  IntegratorVariant=Disabled  SatVariant=Disabled  AWVariant=Disabled  PCopyVariant=Disabled  TRVariant=Disabled  FdbkBlocksVariant=Forward  IdealPFdbkVariant=Disabled  SatFdbkVariant=Disabled  DerivativeFilterVariant=ContFilter  NVariant=InternalParameters  NCopyVariant=Disabled  FilterICVariant=InternalICsFilter  IntegratorICVariant=Disabled  ExternalResetVariant=Disabled  TRSumVariant=Passthrough  SumFdbkVariant=Disabled  SumVariant=Sum_PD  TsampFilterVariant=InternalTs  TsampNgainVariant=Passthrough  TsampIntegralVariant=Disabled_SignalSpec  ExternalSaturationOutDataTypeStr=Inherit: Same as second input
  =R_d1 : slpidlib/PID Controller  Controller=PID  Form=Parallel  TimeDomain=Continuous-time  UseExternalTs=off  SampleTime=-1  IntegratorMethod=Forward Euler  FilterMethod=Forward Euler  ControllerParametersSource=internal  P=0.1  I=0  UseKiTs=off  D=0  N=100  UseFilter=on  TunerSelectOption=Transfer Function Based (PID Tuner App)  InitialConditionSource=internal  InitialConditionForIntegrator=0  InitialConditionForFilter=0  DifferentiatorICPrevScaledInput=0  ExternalReset=none  TrackingMode=off  Kt=1  LimitOutput=off  SatLimitsSource=internal  UpperSaturationLimit=inf  LowerSaturationLimit=-inf  LinearizeAsGain=on  AntiWindupMode=none  Kb=1  LimitIntegrator=off  UpperIntegratorSaturationLimit=inf  LowerIntegratorSaturationLimit=-inf  POutMin=[]  POutMax=[]  IOutMin=[]  IOutMax=[]  DOutMin=[]  DOutMax=[]  NOutMin=[]  NOutMax=[]  SumOutMin=[]  SumOutMax=[]  SaturationOutMin=[]  SaturationOutMax=[]  PParamMin=[]  PParamMax=[]  IParamMin=[]  IParamMax=[]  DParamMin=[]  DParamMax=[]  NParamMin=[]  NParamMax=[]  KbParamMin=[]  KbParamMax=[]  KtParamMin=[]  KtParamMax=[]  KbOutMin=[]  KbOutMax=[]  KtOutMin=[]  KtOutMax=[]  IntegratorOutMin=[]  IntegratorOutMax=[]  FilterOutMin=[]  FilterOutMax=[]  SumI1OutMin=[]  SumI1OutMax=[]  SumI2OutMin=[]  SumI2OutMax=[]  SumI3OutMin=[]  SumI3OutMax=[]  SumI4OutMin=[]  SumI4OutMax=[]  SumDOutMin=[]  SumDOutMax=[]  DifferentiatorOutMin=[]  DifferentiatorOutMax=[]  FilterDiffOutCoefMin=[]  FilterDiffOutCoefMax=[]  ReciprocalOutMin=[]  ReciprocalOutMax=[]  SumDenOutMin=[]  SumDenOutMax=[]  SumNumOutMin=[]  SumNumOutMax=[]  DivideOutMin=[]  DivideOutMax=[]  UdiffTsProdOutMin=[]  UdiffTsProdOutMax=[]  NTsProdOutMin=[]  NTsProdOutMax=[]  UintegralTsProdOutMin=[]  UintegralTsProdOutMax=[]  UngainTsProdOutMin=[]  UngainTsProdOutMax=[]  ClampingZeroOutDataTypeStr=Inherit: Inherit via back propagation  ClampingZeroOutMin=[]  ClampingZeroOutMax=[]  FilterDenConstantOutDataTypeStr=Inherit: Inherit via back propagation  FilterDenConstantOutMin=[]  FilterDenConstantOutMax=[]  PCopyOutDataTypeStr=Inherit: Inherit via back propagation  PCopyOutMin=[]  PCopyOutMax=[]  NCopyOutDataTypeStr=Inherit: Inherit via back propagation  NCopyOutMin=[]  NCopyOutMax=[]  IntegratorContinuousStateAttributes=''  IntegratorStateMustResolveToSignalObject=off  IntegratorRTWStateStorageClass=Auto  FilterContinuousStateAttributes=''  FilterStateMustResolveToSignalObject=off  FilterRTWStateStorageClass=Auto  ParallelPVariant=InternalParameters  IdealPVariant=Disabled  IVariant=InternalParameters  DVariant=InternalParameters  IntegratorVariant=Continuous  SatVariant=Disabled  AWVariant=Passthrough  PCopyVariant=Disabled  TRVariant=Disabled  FdbkBlocksVariant=Forward  IdealPFdbkVariant=Disabled  SatFdbkVariant=Disabled  DerivativeFilterVariant=ContFilter  NVariant=InternalParameters  NCopyVariant=Disabled  FilterICVariant=InternalICsFilter  IntegratorICVariant=InternalICs  ExternalResetVariant=Disabled  TRSumVariant=Passthrough  SumFdbkVariant=Disabled  SumVariant=Sum_PID  TsampFilterVariant=InternalTs  TsampNgainVariant=Passthrough  TsampIntegralVariant=Passthrough  ExternalSaturationOutDataTypeStr=Inherit: Same as second input
  "=dot{ω^b}_d" : slpidlib/PID Controller  Commented=on  Controller=PID  Form=Parallel  TimeDomain=Continuous-time  UseExternalTs=off  SampleTime=-1  IntegratorMethod=Forward Euler  FilterMethod=Forward Euler  ControllerParametersSource=internal  P=[1;1;1]  I=[1;1;1]  UseKiTs=off  D=[1;1;1]  N=100  UseFilter=on  TunerSelectOption=Transfer Function Based (PID Tuner App)  InitialConditionSource=internal  InitialConditionForIntegrator=0  InitialConditionForFilter=0  DifferentiatorICPrevScaledInput=0  ExternalReset=none  TrackingMode=off  Kt=1  LimitOutput=off  SatLimitsSource=internal  UpperSaturationLimit=inf  LowerSaturationLimit=-inf  LinearizeAsGain=on  AntiWindupMode=none  Kb=1  LimitIntegrator=off  UpperIntegratorSaturationLimit=inf  LowerIntegratorSaturationLimit=-inf  POutMin=[]  POutMax=[]  IOutMin=[]  IOutMax=[]  DOutMin=[]  DOutMax=[]  NOutMin=[]  NOutMax=[]  SumOutMin=[]  SumOutMax=[]  SaturationOutMin=[]  SaturationOutMax=[]  PParamMin=[]  PParamMax=[]  IParamMin=[]  IParamMax=[]  DParamMin=[]  DParamMax=[]  NParamMin=[]  NParamMax=[]  KbParamMin=[]  KbParamMax=[]  KtParamMin=[]  KtParamMax=[]  KbOutMin=[]  KbOutMax=[]  KtOutMin=[]  KtOutMax=[]  IntegratorOutMin=[]  IntegratorOutMax=[]  FilterOutMin=[]  FilterOutMax=[]  SumI1OutMin=[]  SumI1OutMax=[]  SumI2OutMin=[]  SumI2OutMax=[]  SumI3OutMin=[]  SumI3OutMax=[]  SumI4OutMin=[]  SumI4OutMax=[]  SumDOutMin=[]  SumDOutMax=[]  DifferentiatorOutMin=[]  DifferentiatorOutMax=[]  FilterDiffOutCoefMin=[]  FilterDiffOutCoefMax=[]  ReciprocalOutMin=[]  ReciprocalOutMax=[]  SumDenOutMin=[]  SumDenOutMax=[]  SumNumOutMin=[]  SumNumOutMax=[]  DivideOutMin=[]  DivideOutMax=[]  UdiffTsProdOutMin=[]  UdiffTsProdOutMax=[]  NTsProdOutMin=[]  NTsProdOutMax=[]  UintegralTsProdOutMin=[]  UintegralTsProdOutMax=[]  UngainTsProdOutMin=[]  UngainTsProdOutMax=[]  ClampingZeroOutDataTypeStr=Inherit: Inherit via back propagation  ClampingZeroOutMin=[]  ClampingZeroOutMax=[]  FilterDenConstantOutDataTypeStr=Inherit: Inherit via back propagation  FilterDenConstantOutMin=[]  FilterDenConstantOutMax=[]  PCopyOutDataTypeStr=Inherit: Inherit via back propagation  PCopyOutMin=[]  PCopyOutMax=[]  NCopyOutDataTypeStr=Inherit: Inherit via back propagation  NCopyOutMin=[]  NCopyOutMax=[]  IntegratorContinuousStateAttributes=''  IntegratorStateMustResolveToSignalObject=off  IntegratorRTWStateStorageClass=Auto  FilterContinuousStateAttributes=''  FilterStateMustResolveToSignalObject=off  FilterRTWStateStorageClass=Auto  ParallelPVariant=InternalParameters  IdealPVariant=Disabled  IVariant=InternalParameters  DVariant=InternalParameters  IntegratorVariant=Continuous  SatVariant=Disabled  AWVariant=Passthrough  PCopyVariant=Disabled  TRVariant=Disabled  FdbkBlocksVariant=Forward  IdealPFdbkVariant=Disabled  SatFdbkVariant=Disabled  DerivativeFilterVariant=ContFilter  NVariant=InternalParameters  NCopyVariant=Disabled  FilterICVariant=InternalICsFilter  IntegratorICVariant=InternalICs  ExternalResetVariant=Disabled  TRSumVariant=Passthrough  SumFdbkVariant=Disabled  SumVariant=Sum_PID  TsampFilterVariant=InternalTs  TsampNgainVariant=Passthrough  TsampIntegralVariant=Passthrough  ExternalSaturationOutDataTypeStr=Inherit: Same as second input
  Gain : Gain  Gain=innertia  Multiplication=Matrix(K*u)
  Matrix Concatenate : Concatenate  NumInputs=3  Mode=Multidimensional array
  Matrix Concatenate1 : Concatenate  NumInputs=3  Mode=Multidimensional array
  Multiport Selector : dspindex/Multiport Selector  rowsOrCols=Rows  idxCellArray={1,2,3}  idxErrMode=Clip Index
  Multiport Selector1 : dspindex/Multiport Selector  rowsOrCols=Rows  idxCellArray={1,2,3}  idxErrMode=Clip Index
  Mux : Mux  Inputs=3
  Mux1 : Mux  Inputs=3
  Reshape1 : Reshape  OutputDimensionality=Column vector (2-D)
  Reshape4 : Reshape  OutputDimensionality=Column vector (2-D)
  Saturation : Saturate  UpperLimit=0.5*pi  LowerLimit=-0.5*pi  ZeroCross=off
      settings: AttributesFormatString=期望角速度限幅
  Saturation1 : Saturate  UpperLimit=0.5e-2 *pi  LowerLimit=-0.5e-2 *pi  ZeroCross=off
      settings: AttributesFormatString=期望角速度限幅
  Scope : Scope
  "e_{\\Theta}" : Sum  Inputs=+-
  "e_{ω^b}" : Sum  Inputs=+-
  mod : Subsystem  mask{a=-pi, b=pi}
      mask DialogControl ParameterGroupVar Prompt: 参数
  tau_d (3,1) : Outport
  wires:
  θ_d (1,1)/1 -> Mux/2
  φ_d (1,1)/1 -> Mux/1
  ψ_d (1,1)/1 -> Mux/3
  Matrix Concatenate1/1 -> Saturation1/1
  Multiport Selector1/3 -> =R_d1/1
  Multiport Selector1/1 -> =P_d1/1
  φ (1,1)/1 -> Mux1/1
  "e_{\\Theta}"/1 -> Scope/1, mod/1(x)
  θ (1,1)/1 -> Mux1/2
  Mux1/1 -> "e_{\\Theta}"/2
  ψ (1,1)/1 -> Mux1/3
  Mux/1 -> "e_{\\Theta}"/1
  Multiport Selector1/2 -> =Q_d1/1
  mod/1(x mod [a,b)) -> Reshape1/1
  Reshape1/1 -> Multiport Selector/1
  =Q_d/1 -> Matrix Concatenate/2
  Multiport Selector/3 -> =R_d/1
  Multiport Selector/1 -> =P_d/1
  "e_{ω^b}"/1 -> Multiport Selector1/1, "=dot{ω^b}_d"/1
  Multiport Selector/2 -> =Q_d/1
  =P_d/1 -> Matrix Concatenate/1
  =R_d/1 -> Matrix Concatenate/3
  Matrix Concatenate/1 -> Saturation/1
  ω^b (3,1)/1 -> Reshape4/1
  Saturation/1 -> "e_{ω^b}"/1
  Reshape4/1 -> "e_{ω^b}"/2
  =P_d1/1 -> Matrix Concatenate1/1
  =Q_d1/1 -> Matrix Concatenate1/2
  =R_d1/1 -> Matrix Concatenate1/3
  Saturation1/1 -> Gain/1
  Gain/1 -> tau_d (3,1)/1

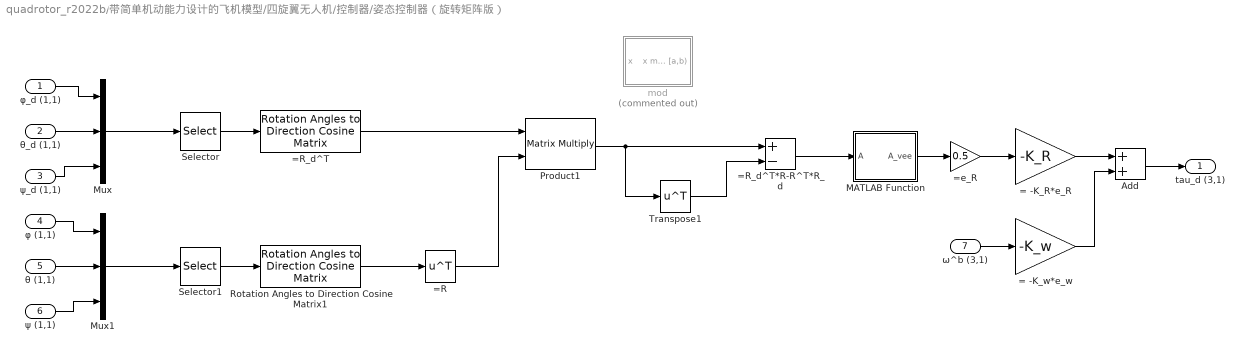
== system quadrotor_r2022b/带简单机动能力设计的飞机模型/四旋翼无人机/控制器/姿态控制器（旋转矩阵版） ==
  φ_d (1,1) : Inport
  θ_d (1,1) : Inport  Port=2
  ψ_d (1,1) : Inport  Port=3
  φ (1,1) : Inport  Port=4
  θ (1,1) : Inport  Port=5
  ψ (1,1) : Inport  Port=6
  ω^b (3,1) : Inport  Port=7
  = -K_R*e_R : Gain  Gain=-K_R
  = -K_w*e_w : Gain  Gain=-K_w
  =R : Math  Operator=transpose
  =R_d^T : sharedtransform/Rotation Angles to Direction Cosine Matrix  rotationOrder=ZYX  aMode=aMode
  =R_d^T*R-R^T*R_d : Sum  Inputs=+-
  =e_R : Gain  Gain=0.5
  Add : Sum
  MATLAB Function : MATLAB Function  TreatAsAtomicUnit=on
  Mux : Mux  Inputs=3
  Mux1 : Mux  Inputs=3
  Product1 : Product  Multiplication=Matrix(*)
  Rotation Angles to Direction Cosine Matrix1 : sharedtransform/Rotation Angles to Direction Cosine Matrix  rotationOrder=ZYX  aMode=aMode
  Selector : Selector  InputPortWidth=3  IndexOptions=Index vector (dialog)  Indices=[3,2,1]  OutputSizes=1
  Selector1 : Selector  InputPortWidth=3  IndexOptions=Index vector (dialog)  Indices=[3,2,1]  OutputSizes=1
  Transpose1 : Math  Operator=transpose
  mod : Subsystem  Commented=on  mask{a=-pi, b=pi}
      mask DialogControl ParameterGroupVar Prompt: 参数
  tau_d (3,1) : Outport
  wires:
  ψ (1,1)/1 -> Mux1/3
  θ (1,1)/1 -> Mux1/2
  φ (1,1)/1 -> Mux1/1
  Product1/1 -> Transpose1/1, =R_d^T*R-R^T*R_d/1
  ψ_d (1,1)/1 -> Mux/3
  θ_d (1,1)/1 -> Mux/2
  φ_d (1,1)/1 -> Mux/1
  Mux1/1 -> Selector1/1
  Mux/1 -> Selector/1
  =R_d^T*R-R^T*R_d/1 -> MATLAB Function/1(A)
  Selector1/1 -> Rotation Angles to Direction Cosine Matrix1/1
  Selector/1 -> =R_d^T/1
  Rotation Angles to Direction Cosine Matrix1/1 -> =R/1
  =R_d^T/1 -> Product1/1
  =R/1 -> Product1/2
  MATLAB Function/1(A_vee) -> =e_R/1
  =e_R/1 -> = -K_R*e_R/1
  ω^b (3,1)/1 -> = -K_w*e_w/1
  = -K_R*e_R/1 -> Add/1
  Add/1 -> tau_d (3,1)/1
  = -K_w*e_w/1 -> Add/2
  Transpose1/1 -> =R_d^T*R-R^T*R_d/2

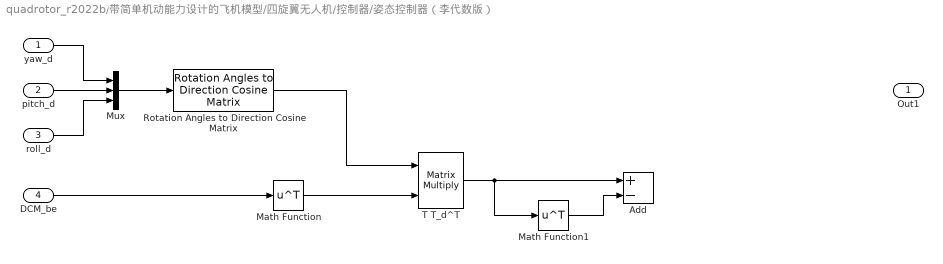
== system quadrotor_r2022b/带简单机动能力设计的飞机模型/四旋翼无人机/控制器/姿态控制器（李代数版） ==
  yaw_d : Inport  PortDimensions=nw
  pitch_d : Inport  Port=2  PortDimensions=nw
  roll_d : Inport  Port=3  PortDimensions=nw
  DCM_be : Inport  Port=4  PortDimensions=nw
  Add : Sum  Inputs=+-
  Math Function : Math  Operator=transpose
  Math Function1 : Math  Operator=transpose
  Mux : Mux  Inputs=3
  Rotation Angles to Direction Cosine Matrix : sharedtransform/Rotation Angles to Direction Cosine Matrix  rotationOrder=ZYX  aMode=aMode
  T T_d^T : Product  Multiplication=Matrix(*)
  Out1 : Outport
  wires:
  yaw_d/1 -> Mux/1
  pitch_d/1 -> Mux/2
  roll_d/1 -> Mux/3
  Mux/1 -> Rotation Angles to Direction Cosine Matrix/1
  Rotation Angles to Direction Cosine Matrix/1 -> T T_d^T/1
  DCM_be/1 -> Math Function/1
  Math Function/1 -> T T_d^T/2
  T T_d^T/1 -> Add/1, Math Function1/1
  Math Function1/1 -> Add/2
